simulink model "testerdoESU2"  (R2022b)
settings: Solver=VariableStepAuto  StartTime=0.0  StopTime=10  RelTol=1e-3
values from neighbouring files (symbols this model uses):
  Ba = -1    [dane.m]    (also in tester23.m; wykresownik33.m; wykresownik35.m; wykresownik36.m)
  Bf = [0.00436 0.00065 0.0119210 0.0127548 0.007765]*10000    [dane.m]    (also in tester23.m = [0.00436 0.00065 1.19210 1.27548 0.007765]; wykresownik33.m = [0.00436 0.00065 1.19210 1.27548 0.007765]; wykresownik35.m = [0.00436 0.00065 1.19210 1.27548 0.007765]; wykresownik36.m = [0.00436 0.00065 1.19210 1.27548 0.007765])
  Bp = -0.3375*5    (= -1.6875)    [dane.m]    (also in tester23.m = 0.3375; wykresownik33.m = -0.3375; wykresownik35.m = -0.3375; wykresownik36.m = -0.3375)
  Bv = -[-0.149 0.181]/1000    [dane.m]    (also in tester23.m = [-0.149 0.181]; wykresownik33.m = [-0.149 0.181]; wykresownik35.m = [-0.149 0.181]; wykresownik36.m = [-0.149 0.181])
  matrixA = table2array(matrixA(:,2:10))    [dane.m]    (also in tester23.m; wykresownik33.m; wykresownik35.m; wykresownik36.m)
settings Model: Creator=48519  LastModifiedBy=48519
settings ModelReferenceCC: EnableRefExpFcnMdlSchedulingChecks=on

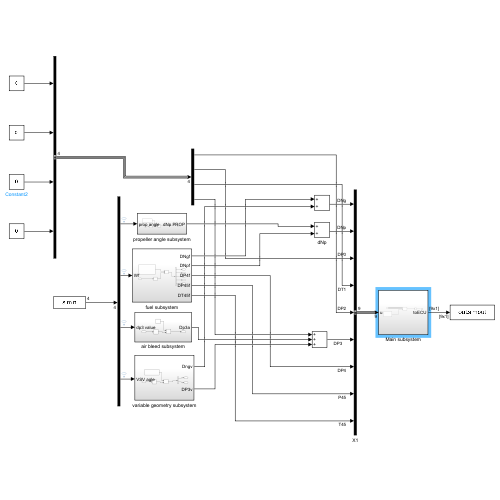
[thumbnail: Simulink's stored preview of the top-level diagram]
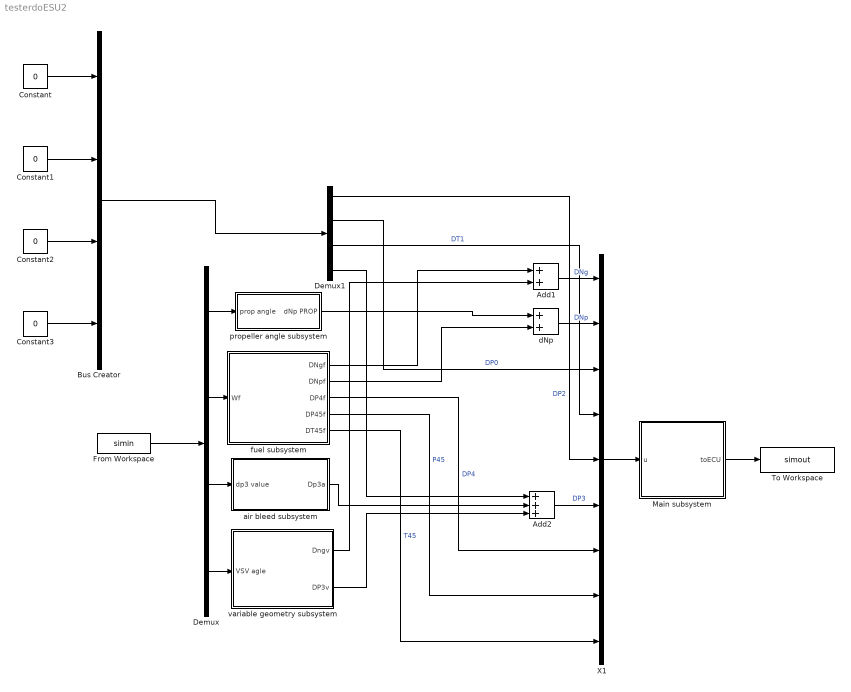
== system testerdoESU2 ==
  Add1 : Sum
  Add2 : Sum  Inputs=+++
  Bus Creator : BusCreator  Inputs=4
  Constant{,1..3} (4 alike) : Constant  Value=0
  Demux : Demux
  Demux1 : Demux
  From Workspace : FromWorkspace  VariableName=simin
  Main subsystem : Subsystem
  To Workspace : ToWorkspace  VariableName=simout  SaveFormat=Timeseries  SampleTime=0.001
  X1 : BusCreator  Inputs=9
  air bleed subsystem : Subsystem
  dNp : Sum
  fuel subsystem : Subsystem
  propeller angle subsystem : Subsystem
  variable geometry subsystem : Subsystem
  wires:
  fuel subsystem/1(DNgf) -> Add1/1
  Demux1/4 -> Add2/1
  Demux1/1 -> X1/5  "DP2"
  Bus Creator/1 -> Demux1/1
  Demux/3 -> air bleed subsystem/1(dp3 value)
  Demux/1 -> propeller angle subsystem/1(prop angle)
  dNp/1 -> X1/2  "DNp"
  Demux/2 -> fuel subsystem/1(Wf)
  propeller angle subsystem/1(dNp PROP) -> dNp/1
  variable geometry subsystem/1(Dngv) -> Add1/2
  Add1/1 -> X1/1  "DNg"
  Demux1/2 -> X1/3  "DP0"
  fuel subsystem/5(DT45f) -> X1/9  "T45"
  Demux1/3 -> X1/4  "DT1"
  Add2/1 -> X1/6  "DP3"
  variable geometry subsystem/2(DP3v) -> Add2/3
  fuel subsystem/4(DP45f) -> X1/8  "P45"
  air bleed subsystem/1(Dp3a) -> Add2/2
  fuel subsystem/3(DP4f) -> X1/7  "DP4"
  Demux/4 -> variable geometry subsystem/1("VSV agle ")
  fuel subsystem/2(DNpf) -> dNp/2
  Constant/1 -> Bus Creator/1
  Constant1/1 -> Bus Creator/2
  Constant3/1 -> Bus Creator/4
  Constant2/1 -> Bus Creator/3
  From Workspace/1 -> Demux/1
  X1/1 -> Main subsystem/1(u)
  Main subsystem/1(toECU) -> To Workspace/1

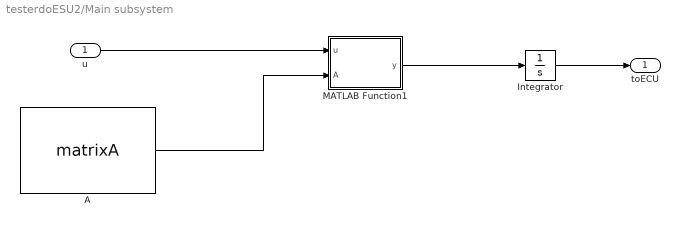
== system testerdoESU2/Main subsystem ==
  u : Inport
  A : Constant  Value=matrixA
  Integrator : Integrator  InitialCondition=1
  MATLAB Function1 : MATLAB Function  TreatAsAtomicUnit=on
  toECU : Outport
  wires:
  u/1 -> MATLAB Function1/1(u)
  MATLAB Function1/1(y) -> Integrator/1
  Integrator/1 -> toECU/1
  A/1 -> MATLAB Function1/2(A)

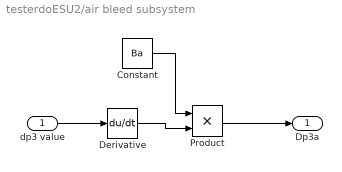
== system testerdoESU2/air bleed subsystem ==
  dp3 value : Inport
  Constant : Constant  Value=Ba
  Derivative : Derivative
  Product : Product
  Dp3a : Outport
  wires:
  Product/1 -> Dp3a/1
  Derivative/1 -> Product/2
  dp3 value/1 -> Derivative/1
  Constant/1 -> Product/1

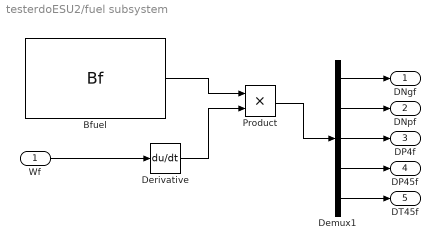
== system testerdoESU2/fuel subsystem ==
  Wf : Inport
  Bfuel : Constant  Value=Bf
  Demux1 : Demux  Outputs=5
  Derivative : Derivative
  Product : Product
  DNgf : Outport
  DNpf : Outport  Port=2
  DP4f : Outport  Port=3
  DP45f : Outport  Port=4
  DT45f : Outport  Port=5
  wires:
  Product/1 -> Demux1/1
  Bfuel/1 -> Product/1
  Wf/1 -> Derivative/1
  Derivative/1 -> Product/2
  Demux1/4 -> DP45f/1
  Demux1/1 -> DNgf/1
  Demux1/2 -> DNpf/1
  Demux1/3 -> DP4f/1
  Demux1/5 -> DT45f/1

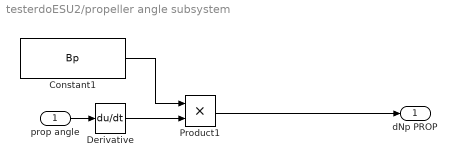
== system testerdoESU2/propeller angle subsystem ==
  prop angle : Inport
  Constant1 : Constant  Value=Bp
  Derivative : Derivative
  Product1 : Product
  dNp PROP : Outport
  wires:
  prop angle/1 -> Derivative/1
  Constant1/1 -> Product1/1
  Derivative/1 -> Product1/2
  Product1/1 -> dNp PROP/1

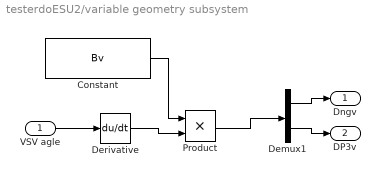
== system testerdoESU2/variable geometry subsystem ==
  "VSV agle " : Inport
  Constant : Constant  Value=Bv
  Demux1 : Demux  Outputs=2
  Derivative : Derivative
  Product : Product
  Dngv : Outport
  DP3v : Outport  Port=2
  wires:
  Constant/1 -> Product/1
  "VSV agle "/1 -> Derivative/1
  Product/1 -> Demux1/1
  Demux1/2 -> DP3v/1
  Demux1/1 -> Dngv/1
  Derivative/1 -> Product/2

== matlab function testerdoESU2/Main subsystem/MATLAB Function1 ==
  data: u input; y output; A input
function y = fcn(u,A)
starter=max(abs(u));
maxer=starter;
[x]=find(abs(u)==maxer,1,"first");
k= x(1,1);
i=0;
while (maxer>0.25) && (i<100)
    u=u+A*u;
    u=u+A*u;
    maxer= abs((abs(u(k))-starter))/(starter+0.1);
    i=i+1;
end
    y=u;
